simulink library "ECO_TestLibs"  (R2018a)
settings: Solver=ode45  StartTime=0.0  StopTime=10.0  RelTol=1e-3  EnableMultiTasking=on
undefined symbols (not defined in the file or in its folder): h, km
libraries: CoderSF_BSW_Libs x643, $bdroot x217, SF_CanService_Libs x60, simulink x12
(part 7 of 7)

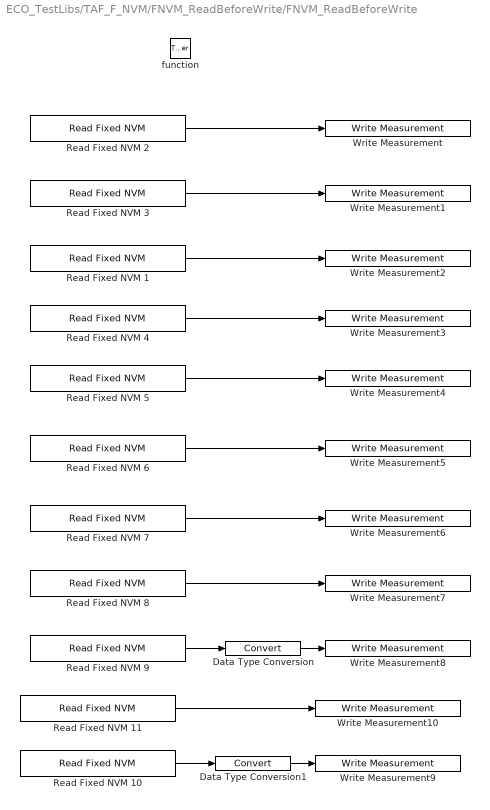
== system ECO_TestLibs/TAF_F_NVM/FNVM_ReadBeforeWrite/FNVM_ReadBeforeWrite ==
  function : TriggerPort  TriggerType=function-call  VariantControl=(inherit)
  Data Type Conversion : DataTypeConversion
  Data Type Conversion1 : DataTypeConversion
  Read Fixed NVM 1 : CoderSF_BSW_Libs/Non-volatile Memory Blocks/Read Fixed NVM   data_name=Fnvm_single
      settings: SourceProductName=EcoCoder Blocks
  Read Fixed NVM 10 : CoderSF_BSW_Libs/Non-volatile Memory Blocks/Read Fixed NVM   data_name=Fnvm_double2
      settings: SourceProductName=EcoCoder Blocks
  Read Fixed NVM 11 : CoderSF_BSW_Libs/Non-volatile Memory Blocks/Read Fixed NVM   data_name=Fnvm_single2
      settings: SourceProductName=EcoCoder Blocks
  Read Fixed NVM 2 : CoderSF_BSW_Libs/Non-volatile Memory Blocks/Read Fixed NVM   data_name=Fnvm_int32
      settings: SourceProductName=EcoCoder Blocks
  Read Fixed NVM 3 : CoderSF_BSW_Libs/Non-volatile Memory Blocks/Read Fixed NVM   data_name=Fnvm_uint32
      settings: SourceProductName=EcoCoder Blocks
  Read Fixed NVM 4 : CoderSF_BSW_Libs/Non-volatile Memory Blocks/Read Fixed NVM   data_name=Fnvm_int16
      settings: SourceProductName=EcoCoder Blocks
  Read Fixed NVM 5 : CoderSF_BSW_Libs/Non-volatile Memory Blocks/Read Fixed NVM   data_name=Fnvm_uint16
      settings: SourceProductName=EcoCoder Blocks
  Read Fixed NVM 6 : CoderSF_BSW_Libs/Non-volatile Memory Blocks/Read Fixed NVM   data_name=Fnvm_boolean
      settings: SourceProductName=EcoCoder Blocks
  Read Fixed NVM 7 : CoderSF_BSW_Libs/Non-volatile Memory Blocks/Read Fixed NVM   data_name=Fnvm_uint8
      settings: SourceProductName=EcoCoder Blocks
  Read Fixed NVM 8 : CoderSF_BSW_Libs/Non-volatile Memory Blocks/Read Fixed NVM   data_name=Fnvm_int8
      settings: SourceProductName=EcoCoder Blocks
  Read Fixed NVM 9 : CoderSF_BSW_Libs/Non-volatile Memory Blocks/Read Fixed NVM   data_name=Fnvm_double
      settings: SourceProductName=EcoCoder Blocks
  Write Measurement : CoderSF_BSW_Libs/Calibration & Measurement/Write Measurement  variable_name=Fnvm_int32Init  variable_value=0  variable_type=int32  numD=1  unitStr=""  descStr=""
      settings: AttributesFormatString=value:%<variable_value> type:%<variable_type>  SourceProductName=EcoCoder Blocks
  Write Measurement1 : CoderSF_BSW_Libs/Calibration & Measurement/Write Measurement  variable_name=Fnvm_uint32Init  variable_value=0  variable_type=uint32  numD=4  unitStr=""  descStr=""
      settings: AttributesFormatString=value:%<variable_value> type:%<variable_type>  SourceProductName=EcoCoder Blocks
  Write Measurement10 : CoderSF_BSW_Libs/Calibration & Measurement/Write Measurement  variable_name=Fnvm_single2Init  variable_value=0  variable_type=single  numD=1  unitStr=""  descStr=""
      settings: AttributesFormatString=value:%<variable_value> type:%<variable_type>  SourceProductName=EcoCoder Blocks
  Write Measurement2 : CoderSF_BSW_Libs/Calibration & Measurement/Write Measurement  variable_name=Fnvm_singleInit  variable_value=0  variable_type=single  numD=1  unitStr=""  descStr=""
      settings: AttributesFormatString=value:%<variable_value> type:%<variable_type>  SourceProductName=EcoCoder Blocks
  Write Measurement3 : CoderSF_BSW_Libs/Calibration & Measurement/Write Measurement  variable_name=Fnvm_int16Init  variable_value=0  variable_type=int16  numD=2  unitStr=""  descStr=""
      settings: AttributesFormatString=value:%<variable_value> type:%<variable_type>  SourceProductName=EcoCoder Blocks
  Write Measurement4 : CoderSF_BSW_Libs/Calibration & Measurement/Write Measurement  variable_name=Fnvm_uint16Init  variable_value=0  variable_type=uint16  numD=2  unitStr=""  descStr=""
      settings: AttributesFormatString=value:%<variable_value> type:%<variable_type>  SourceProductName=EcoCoder Blocks
  Write Measurement5 : CoderSF_BSW_Libs/Calibration & Measurement/Write Measurement  variable_name=Fnvm_booleanInit  variable_value=0  variable_type=boolean  numD=4  unitStr=""  descStr=""
      settings: AttributesFormatString=value:%<variable_value> type:%<variable_type>  SourceProductName=EcoCoder Blocks
  Write Measurement6 : CoderSF_BSW_Libs/Calibration & Measurement/Write Measurement  variable_name=Fnvm_uint8Init  variable_value=0  variable_type=uint8  numD=1  unitStr=""  descStr=""
      settings: AttributesFormatString=value:%<variable_value> type:%<variable_type>  SourceProductName=EcoCoder Blocks
  Write Measurement7 : CoderSF_BSW_Libs/Calibration & Measurement/Write Measurement  variable_name=Fnvm_int8Init  variable_value=0  variable_type=int8  numD=2  unitStr=""  descStr=""
      settings: AttributesFormatString=value:%<variable_value> type:%<variable_type>  SourceProductName=EcoCoder Blocks
  Write Measurement8 : CoderSF_BSW_Libs/Calibration & Measurement/Write Measurement  variable_name=Fnvm_doubleInit  variable_value=0  variable_type=single  numD=1  unitStr=""  descStr=""
      settings: AttributesFormatString=value:%<variable_value> type:%<variable_type>  SourceProductName=EcoCoder Blocks
  Write Measurement9 : CoderSF_BSW_Libs/Calibration & Measurement/Write Measurement  variable_name=Fnvm_double2Init  variable_value=0  variable_type=single  numD=1  unitStr=""  descStr=""
      settings: AttributesFormatString=value:%<variable_value> type:%<variable_type>  SourceProductName=EcoCoder Blocks
  wires:
  Read Fixed NVM 8/1 -> Write Measurement7/1
  Read Fixed NVM 6/1 -> Write Measurement5/1
  Read Fixed NVM 5/1 -> Write Measurement4/1
  Read Fixed NVM 1/1 -> Write Measurement2/1
  Read Fixed NVM 9/1 -> Data Type Conversion/1
  Read Fixed NVM 3/1 -> Write Measurement1/1
  Read Fixed NVM 4/1 -> Write Measurement3/1
  Data Type Conversion/1 -> Write Measurement8/1
  Read Fixed NVM 2/1 -> Write Measurement/1
  Read Fixed NVM 7/1 -> Write Measurement6/1
  Read Fixed NVM 10/1 -> Data Type Conversion1/1
  Data Type Conversion1/1 -> Write Measurement9/1
  Read Fixed NVM 11/1 -> Write Measurement10/1

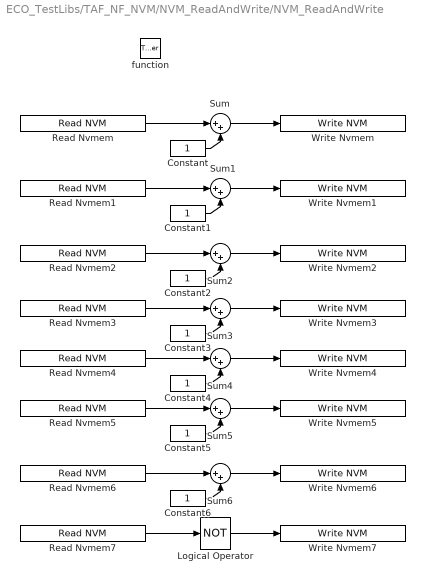
== system ECO_TestLibs/TAF_NF_NVM/NVM_ReadAndWrite/NVM_ReadAndWrite ==
  function : TriggerPort  TriggerType=function-call  VariantControl=(inherit)
  Constant{,1..6} (7 alike) : Constant  OutDataTypeStr=Inherit: Inherit via back propagation  SampleTime=-1
  Logical Operator : Logic  Operator=NOT  AllPortsSameDT=off  OutDataTypeStr=boolean
  Read Nvmem : CoderSF_BSW_Libs/Non-volatile Memory Blocks/Read NVM  variable_name=ASW_Nvm_single  variable_type=Inherit from 'Variable definition'
      settings: AttributesFormatString=type:%<variable_type>  SourceProductName=EcoCoder Blocks
  Read Nvmem1 : CoderSF_BSW_Libs/Non-volatile Memory Blocks/Read NVM  variable_name=ASW_Nvm_int8  variable_type=Inherit from 'Variable definition'
      settings: AttributesFormatString=type:%<variable_type>  SourceProductName=EcoCoder Blocks
  Read Nvmem2 : CoderSF_BSW_Libs/Non-volatile Memory Blocks/Read NVM  variable_name=ASW_Nvm_uint8  variable_type=Inherit from 'Variable definition'
      settings: AttributesFormatString=type:%<variable_type>  SourceProductName=EcoCoder Blocks
  Read Nvmem3 : CoderSF_BSW_Libs/Non-volatile Memory Blocks/Read NVM  variable_name=ASW_Nvm_int16  variable_type=Inherit from 'Variable definition'
      settings: AttributesFormatString=type:%<variable_type>  SourceProductName=EcoCoder Blocks
  Read Nvmem4 : CoderSF_BSW_Libs/Non-volatile Memory Blocks/Read NVM  variable_name=ASW_Nvm_uint16  variable_type=Inherit from 'Variable definition'
      settings: AttributesFormatString=type:%<variable_type>  SourceProductName=EcoCoder Blocks
  Read Nvmem5 : CoderSF_BSW_Libs/Non-volatile Memory Blocks/Read NVM  variable_name=ASW_Nvm_int32  variable_type=Inherit from 'Variable definition'
      settings: AttributesFormatString=type:%<variable_type>  SourceProductName=EcoCoder Blocks
  Read Nvmem6 : CoderSF_BSW_Libs/Non-volatile Memory Blocks/Read NVM  variable_name=ASW_Nvm_uint32  variable_type=Inherit from 'Variable definition'
      settings: AttributesFormatString=type:%<variable_type>  SourceProductName=EcoCoder Blocks
  Read Nvmem7 : CoderSF_BSW_Libs/Non-volatile Memory Blocks/Read NVM  variable_name=ASW_Nvm_boolean  variable_type=Inherit from 'Variable definition'
      settings: AttributesFormatString=type:%<variable_type>  SourceProductName=EcoCoder Blocks
  Sum{,1..6} (7 alike) : Sum  Inputs=|++
  Write Nvmem : CoderSF_BSW_Libs/Non-volatile Memory Blocks/Write NVM  variable_name=ASW_Nvm_single  flgDef=on  variable_value=2  variable_type=single  variable_numD=1  unitStr=""  descStr=""  EcoCoderBlockID=N001_NVMVDEF
      settings: AttributesFormatString=value:%<variable_value> type:%<variable_type> D:%<variable_numD>  SourceProductName=EcoCoder Blocks
  Write Nvmem1 : CoderSF_BSW_Libs/Non-volatile Memory Blocks/Write NVM  variable_name=ASW_Nvm_int8  flgDef=on  variable_value=2  variable_type=int8  variable_numD=1  unitStr=""  descStr=""  EcoCoderBlockID=N001_NVMVDEF
      settings: AttributesFormatString=value:%<variable_value> type:%<variable_type> D:%<variable_numD>  SourceProductName=EcoCoder Blocks
  Write Nvmem2 : CoderSF_BSW_Libs/Non-volatile Memory Blocks/Write NVM  variable_name=ASW_Nvm_uint8  flgDef=on  variable_value=2  variable_type=uint8  variable_numD=1  unitStr=""  descStr=""  EcoCoderBlockID=N001_NVMVDEF
      settings: AttributesFormatString=value:%<variable_value> type:%<variable_type> D:%<variable_numD>  SourceProductName=EcoCoder Blocks
  Write Nvmem3 : CoderSF_BSW_Libs/Non-volatile Memory Blocks/Write NVM  variable_name=ASW_Nvm_int16  flgDef=on  variable_value=2  variable_type=int16  variable_numD=1  unitStr=""  descStr=""  EcoCoderBlockID=N001_NVMVDEF
      settings: AttributesFormatString=value:%<variable_value> type:%<variable_type> D:%<variable_numD>  SourceProductName=EcoCoder Blocks
  Write Nvmem4 : CoderSF_BSW_Libs/Non-volatile Memory Blocks/Write NVM  variable_name=ASW_Nvm_uint16  flgDef=on  variable_value=2  variable_type=uint16  variable_numD=1  unitStr=""  descStr=""  EcoCoderBlockID=N001_NVMVDEF
      settings: AttributesFormatString=value:%<variable_value> type:%<variable_type> D:%<variable_numD>  SourceProductName=EcoCoder Blocks
  Write Nvmem5 : CoderSF_BSW_Libs/Non-volatile Memory Blocks/Write NVM  variable_name=ASW_Nvm_int32  flgDef=on  variable_value=2  variable_type=int32  variable_numD=1  unitStr=""  descStr=""  EcoCoderBlockID=N001_NVMVDEF
      settings: AttributesFormatString=value:%<variable_value> type:%<variable_type> D:%<variable_numD>  SourceProductName=EcoCoder Blocks
  Write Nvmem6 : CoderSF_BSW_Libs/Non-volatile Memory Blocks/Write NVM  variable_name=ASW_Nvm_uint32  flgDef=on  variable_value=2  variable_type=uint32  variable_numD=1  unitStr=""  descStr=""  EcoCoderBlockID=N001_NVMVDEF
      settings: AttributesFormatString=value:%<variable_value> type:%<variable_type> D:%<variable_numD>  SourceProductName=EcoCoder Blocks
  Write Nvmem7 : CoderSF_BSW_Libs/Non-volatile Memory Blocks/Write NVM  variable_name=ASW_Nvm_boolean  flgDef=on  variable_value=0  variable_type=boolean  variable_numD=1  unitStr=""  descStr=""  EcoCoderBlockID=N001_NVMVDEF
      settings: AttributesFormatString=value:%<variable_value> type:%<variable_type> D:%<variable_numD>  SourceProductName=EcoCoder Blocks
  wires:
  Read Nvmem7/1 -> Logical Operator/1
  Logical Operator/1 -> Write Nvmem7/1
  Read Nvmem6/1 -> Sum6/1
  Constant6/1 -> Sum6/2
  Sum6/1 -> Write Nvmem6/1
  Read Nvmem5/1 -> Sum5/1
  Constant5/1 -> Sum5/2
  Sum5/1 -> Write Nvmem5/1
  Read Nvmem4/1 -> Sum4/1
  Constant4/1 -> Sum4/2
  Sum4/1 -> Write Nvmem4/1
  Read Nvmem3/1 -> Sum3/1
  Constant3/1 -> Sum3/2
  Sum3/1 -> Write Nvmem3/1
  Read Nvmem2/1 -> Sum2/1
  Constant2/1 -> Sum2/2
  Sum2/1 -> Write Nvmem2/1
  Read Nvmem1/1 -> Sum1/1
  Constant1/1 -> Sum1/2
  Sum1/1 -> Write Nvmem1/1
  Read Nvmem/1 -> Sum/1
  Constant/1 -> Sum/2
  Sum/1 -> Write Nvmem/1

== system ECO_TestLibs/TAF_NF_NVM/NVM_ReadBeforeWrite/NVM_ReadBeforeWrite ==
  function : TriggerPort  TriggerType=function-call  VariantControl=(inherit)
  Measurement Probe : CoderSF_BSW_Libs/Calibration & Measurement/Write Measurement  variable_name=ASW_V_singleInit  variable_value=0  variable_type=single  numD=1  unitStr=""  descStr=""
      settings: AttributesFormatString=value:%<variable_value> type:%<variable_type>  SourceProductName=EcoCoder Blocks
  Measurement Probe1 : CoderSF_BSW_Libs/Calibration & Measurement/Write Measurement  variable_name=ASW_V_int8Init  variable_value=0  variable_type=int8  numD=1  unitStr=""  descStr=""
      settings: AttributesFormatString=value:%<variable_value> type:%<variable_type>  SourceProductName=EcoCoder Blocks
  Measurement Probe2 : CoderSF_BSW_Libs/Calibration & Measurement/Write Measurement  variable_name=ASW_V_uint8Init  variable_value=0  variable_type=uint8  numD=1  unitStr=""  descStr=""
      settings: AttributesFormatString=value:%<variable_value> type:%<variable_type>  SourceProductName=EcoCoder Blocks
  Measurement Probe3 : CoderSF_BSW_Libs/Calibration & Measurement/Write Measurement  variable_name=ASW_V_int16Init  variable_value=0  variable_type=int16  numD=1  unitStr=""  descStr=""
      settings: AttributesFormatString=value:%<variable_value> type:%<variable_type>  SourceProductName=EcoCoder Blocks
  Measurement Probe4 : CoderSF_BSW_Libs/Calibration & Measurement/Write Measurement  variable_name=ASW_V_uint16Init  variable_value=0  variable_type=uint16  numD=1  unitStr=""  descStr=""
      settings: AttributesFormatString=value:%<variable_value> type:%<variable_type>  SourceProductName=EcoCoder Blocks
  Measurement Probe5 : CoderSF_BSW_Libs/Calibration & Measurement/Write Measurement  variable_name=ASW_V_int32Init  variable_value=0  variable_type=int32  numD=1  unitStr=""  descStr=""
      settings: AttributesFormatString=value:%<variable_value> type:%<variable_type>  SourceProductName=EcoCoder Blocks
  Measurement Probe6 : CoderSF_BSW_Libs/Calibration & Measurement/Write Measurement  variable_name=ASW_V_uint32Init  variable_value=0  variable_type=uint32  numD=1  unitStr=""  descStr=""
      settings: AttributesFormatString=value:%<variable_value> type:%<variable_type>  SourceProductName=EcoCoder Blocks
  Measurement Probe7 : CoderSF_BSW_Libs/Calibration & Measurement/Write Measurement  variable_name=ASW_V_booleanInit  variable_value=0  variable_type=boolean  numD=1  unitStr=""  descStr=""
      settings: AttributesFormatString=value:%<variable_value> type:%<variable_type>  SourceProductName=EcoCoder Blocks
  Read Nvmem : CoderSF_BSW_Libs/Non-volatile Memory Blocks/Read NVM  variable_name=ASW_Nvm_single  variable_type=Inherit from 'Variable definition'
      settings: AttributesFormatString=type:%<variable_type>  SourceProductName=EcoCoder Blocks
  Read Nvmem1 : CoderSF_BSW_Libs/Non-volatile Memory Blocks/Read NVM  variable_name=ASW_Nvm_int8  variable_type=Inherit from 'Variable definition'
      settings: AttributesFormatString=type:%<variable_type>  SourceProductName=EcoCoder Blocks
  Read Nvmem2 : CoderSF_BSW_Libs/Non-volatile Memory Blocks/Read NVM  variable_name=ASW_Nvm_uint8  variable_type=Inherit from 'Variable definition'
      settings: AttributesFormatString=type:%<variable_type>  SourceProductName=EcoCoder Blocks
  Read Nvmem3 : CoderSF_BSW_Libs/Non-volatile Memory Blocks/Read NVM  variable_name=ASW_Nvm_int16  variable_type=Inherit from 'Variable definition'
      settings: AttributesFormatString=type:%<variable_type>  SourceProductName=EcoCoder Blocks
  Read Nvmem4 : CoderSF_BSW_Libs/Non-volatile Memory Blocks/Read NVM  variable_name=ASW_Nvm_uint16  variable_type=Inherit from 'Variable definition'
      settings: AttributesFormatString=type:%<variable_type>  SourceProductName=EcoCoder Blocks
  Read Nvmem5 : CoderSF_BSW_Libs/Non-volatile Memory Blocks/Read NVM  variable_name=ASW_Nvm_int32  variable_type=Inherit from 'Variable definition'
      settings: AttributesFormatString=type:%<variable_type>  SourceProductName=EcoCoder Blocks
  Read Nvmem6 : CoderSF_BSW_Libs/Non-volatile Memory Blocks/Read NVM  variable_name=ASW_Nvm_uint32  variable_type=Inherit from 'Variable definition'
      settings: AttributesFormatString=type:%<variable_type>  SourceProductName=EcoCoder Blocks
  Read Nvmem7 : CoderSF_BSW_Libs/Non-volatile Memory Blocks/Read NVM  variable_name=ASW_Nvm_boolean  variable_type=Inherit from 'Variable definition'
      settings: AttributesFormatString=type:%<variable_type>  SourceProductName=EcoCoder Blocks
  wires:
  Read Nvmem/1 -> Measurement Probe/1
  Read Nvmem1/1 -> Measurement Probe1/1
  Read Nvmem2/1 -> Measurement Probe2/1
  Read Nvmem3/1 -> Measurement Probe3/1
  Read Nvmem4/1 -> Measurement Probe4/1
  Read Nvmem5/1 -> Measurement Probe5/1
  Read Nvmem6/1 -> Measurement Probe6/1
  Read Nvmem7/1 -> Measurement Probe7/1

== system ECO_TestLibs/TAF_NF_NVM/Test_NVMStoreFailed/F_Store_All_NVM_Data ==
  function : TriggerPort  TriggerType=function-call  VariantControl=(inherit)
  Logical Operator : Logic  Operator=NOT  AllPortsSameDT=off  OutDataTypeStr=boolean
  Store All NVM Data : CoderSF_BSW_Libs/Non-volatile Memory Blocks/Store All NVM Data  TriggerTypeSet=rising
      settings: SourceProductName=EcoCoder Blocks
  Unit Delay : UnitDelay  SampleTime=-1
  wires:
  Logical Operator/1 -> Unit Delay/1
  Unit Delay/1 -> Store All NVM Data/Trigger, Logical Operator/1

== system ECO_TestLibs/TAF_SWD/TAF_SWD/Service Software Watchdog ==
  Enable : EnablePort
  Service Software Watchdog : CoderSF_BSW_Libs/System Management Blocks/Service Software Watchdog  EcoCoderBlockID=W001_WDGFeed
      settings: SourceProductName=EcoCoder Blocks

== system ECO_TestLibs/TAF_SYS/Shutdown Power/Enabled Subsystem ==
  Enable : EnablePort
  Read Calibration2 : CoderSF_BSW_Libs/Calibration & Measurement/Read Calibration  variable_name=WKUP_flgPwrDelay_val  variable_value=0  variable_type=boolean  variable_min=[]  variable_max=[]  unitStr=""  descStr=""
      settings: AttributesFormatString=value:%<variable_value> type:%<variable_type> max:%<variable_max> Min:%<variable_min>  SourceProductName=EcoCoder Blocks
  "Switch Internal " : CoderSF_BSW_Libs/Digital I//O/Switch Internal   portNum=PowerDelay
      settings: SourceProductName=EcoCoder Blocks
  Write and Read Measurement2 : CoderSF_BSW_Libs/Calibration & Measurement/Write and Read Measurement  variable_name=WKUP_flgPwrDelay  variable_value=0  variable_type=boolean  numD=1  unitStr=""  descStr=""
      settings: AttributesFormatString=value:%<variable_value> type:%<variable_type>  SourceProductName=EcoCoder Blocks
  wires:
  Read Calibration2/1 -> Write and Read Measurement2/1
  Write and Read Measurement2/1 -> "Switch Internal "/1

== system ECO_TestLibs/TAF_TRI/Test_DeadWhile_H1m/Function-Call Subsystem ==
  In1 : Inport
  function : TriggerPort  TriggerType=function-call  VariantControl=(inherit)
  Out1 : Outport
  wires:
  In1/1 -> Out1/1

== system ECO_TestLibs/TAF_TRI/Test_DeadWhile_L1m/Function-Call Subsystem ==
  In1 : Inport
  function : TriggerPort  TriggerType=function-call  VariantControl=(inherit)
  Out1 : Outport
  wires:
  In1/1 -> Out1/1

== system ECO_TestLibs/LINAMaster/RTX/Delay2/Rising Edge ==
  in : Inport  OutDataTypeStr=boolean
  Logical Operator : Logic  AllPortsSameDT=off  OutDataTypeStr=boolean
  Logical Operator1 : Logic  Operator=NOT  AllPortsSameDT=off  OutDataTypeStr=boolean
  Unit Delay : UnitDelay  InitialCondition=InitialCondition  SampleTime=-1
  out : Outport  OutDataTypeStr=boolean
  wires:
  Logical Operator1/1 -> Logical Operator/2
  Logical Operator/1 -> out/1
  Unit Delay/1 -> Logical Operator1/1
  in/1 -> Unit Delay/1, Logical Operator/1

== system ECO_TestLibs/LINAMaster/RTX/Mst Rx Mod/Subsystem ==
  In1 : Inport
  Trigger : TriggerPort  VariantControl=(inherit)  PortDimensions=1
  Send CAN Data : CoderSF_BSW_Libs/CAN/Send CAN Data  channel=CAN_C  txlen=3  txid=hex2dec('200')  frametype=Standard(11-bit ID)  showerror=off
      settings: SourceProductName=EcoCoder Blocks
  wires:
  In1/1 -> Send CAN Data/1

== system ECO_TestLibs/LINASlave/Rx/Subsystem/cntValue1 ==
  10 : Constant  Value=10  OutDataTypeStr=Inherit: Inherit via back propagation
  5 : Constant  Value=1000000000  OutDataTypeStr=Inherit: Inherit via back propagation
  6 : Constant  OutDataTypeStr=Inherit: Inherit via back propagation
  7 : Constant  Value=10000000  OutDataTypeStr=Inherit: Inherit via back propagation
  8 : Constant  Value=100000  OutDataTypeStr=Inherit: Inherit via back propagation
  9 : Constant  Value=1000  OutDataTypeStr=Inherit: Inherit via back propagation
  Delay : simulink/Discrete/Integer Delay  NumDelays=1  vinit=1  samptime=-1
      settings: SourceProductName=Simulink  SourceProductBaseCode=SL
  Sum : Sum  Inputs=|++
  Terminator : Terminator
  ValueConvert : Subsystem
  ValueConvert1 : Subsystem
  ValueConvert2 : Subsystem
  ValueConvert3 : Subsystem
  ValueConvert4 : Subsystem
  m0 : CoderSF_BSW_Libs/Calibration & Measurement/Write and Read Measurement  variable_name=cnt0  variable_value=0  variable_type=uint32  numD=1  unitStr=""  descStr=""
      settings: AttributesFormatString=type:%<variable_type> Dimensions:%<numD>  SourceProductName=EcoCoder Blocks
  Out1 : Outport
  Out2 : Outport  Port=2
  Out3 : Outport  Port=3
  Out4 : Outport  Port=4
  Out5 : Outport  Port=5
  wires:
  ValueConvert/1(Out1) -> Out1/1
  5/1 -> ValueConvert/2(In2)
  7/1 -> ValueConvert1/2(In2)
  8/1 -> ValueConvert2/2(In2)
  9/1 -> ValueConvert3/2(In2)
  10/1 -> ValueConvert4/2(In2)
  m0/1 -> ValueConvert/1(In1)
  6/1 -> Sum/2
  Delay/1 -> Sum/1, m0/1
  Sum/1 -> Delay/1
  ValueConvert1/1(Out1) -> Out2/1
  ValueConvert/2(Out2) -> ValueConvert1/1(In1)
  ValueConvert1/2(Out2) -> ValueConvert2/1(In1)
  ValueConvert2/1(Out1) -> Out3/1
  ValueConvert2/2(Out2) -> ValueConvert3/1(In1)
  ValueConvert3/1(Out1) -> Out4/1
  ValueConvert3/2(Out2) -> ValueConvert4/1(In1)
  ValueConvert4/1(Out1) -> Out5/1
  ValueConvert4/2(Out2) -> Terminator/1

== system ECO_TestLibs/LINASlave/Rx/Subsystem1/cntValue1 ==
  10 : Constant  Value=10  OutDataTypeStr=Inherit: Inherit via back propagation
  5 : Constant  Value=1000000000  OutDataTypeStr=Inherit: Inherit via back propagation
  6 : Constant  OutDataTypeStr=Inherit: Inherit via back propagation
  7 : Constant  Value=10000000  OutDataTypeStr=Inherit: Inherit via back propagation
  8 : Constant  Value=100000  OutDataTypeStr=Inherit: Inherit via back propagation
  9 : Constant  Value=1000  OutDataTypeStr=Inherit: Inherit via back propagation
  Delay : simulink/Discrete/Integer Delay  NumDelays=1  vinit=1  samptime=-1
      settings: SourceProductName=Simulink  SourceProductBaseCode=SL
  Sum : Sum  Inputs=|++
  Terminator : Terminator
  ValueConvert : Subsystem
  ValueConvert1 : Subsystem
  ValueConvert2 : Subsystem
  ValueConvert3 : Subsystem
  ValueConvert4 : Subsystem
  m0 : CoderSF_BSW_Libs/Calibration & Measurement/Write and Read Measurement  variable_name=cnt1  variable_value=0  variable_type=uint32  numD=1  unitStr=""  descStr=""
      settings: AttributesFormatString=type:%<variable_type> Dimensions:%<numD>  SourceProductName=EcoCoder Blocks
  Out1 : Outport
  Out2 : Outport  Port=2
  Out3 : Outport  Port=3
  Out4 : Outport  Port=4
  Out5 : Outport  Port=5
  wires:
  ValueConvert/1(Out1) -> Out1/1
  5/1 -> ValueConvert/2(In2)
  7/1 -> ValueConvert1/2(In2)
  8/1 -> ValueConvert2/2(In2)
  9/1 -> ValueConvert3/2(In2)
  10/1 -> ValueConvert4/2(In2)
  m0/1 -> ValueConvert/1(In1)
  6/1 -> Sum/2
  Delay/1 -> Sum/1, m0/1
  Sum/1 -> Delay/1
  ValueConvert1/1(Out1) -> Out2/1
  ValueConvert/2(Out2) -> ValueConvert1/1(In1)
  ValueConvert1/2(Out2) -> ValueConvert2/1(In1)
  ValueConvert2/1(Out1) -> Out3/1
  ValueConvert2/2(Out2) -> ValueConvert3/1(In1)
  ValueConvert3/1(Out1) -> Out4/1
  ValueConvert3/2(Out2) -> ValueConvert4/1(In1)
  ValueConvert4/1(Out1) -> Out5/1
  ValueConvert4/2(Out2) -> Terminator/1

== system ECO_TestLibs/LINASlave/Rx/Subsystem2/cntValue ==
  10 : Constant  Value=10  OutDataTypeStr=Inherit: Inherit via back propagation
  5 : Constant  Value=1000000000  OutDataTypeStr=Inherit: Inherit via back propagation
  6 : Constant  OutDataTypeStr=Inherit: Inherit via back propagation
  7 : Constant  Value=10000000  OutDataTypeStr=Inherit: Inherit via back propagation
  8 : Constant  Value=100000  OutDataTypeStr=Inherit: Inherit via back propagation
  9 : Constant  Value=1000  OutDataTypeStr=Inherit: Inherit via back propagation
  Delay : simulink/Discrete/Integer Delay  NumDelays=1  vinit=1  samptime=-1
      settings: SourceProductName=Simulink  SourceProductBaseCode=SL
  Sum : Sum  Inputs=|++
  Terminator : Terminator
  ValueConvert : Subsystem
  ValueConvert1 : Subsystem
  ValueConvert2 : Subsystem
  ValueConvert3 : Subsystem
  ValueConvert4 : Subsystem
  m0 : CoderSF_BSW_Libs/Calibration & Measurement/Write and Read Measurement  variable_name=cnt2  variable_value=0  variable_type=uint32  numD=1  unitStr=""  descStr=""
      settings: AttributesFormatString=type:%<variable_type> Dimensions:%<numD>  SourceProductName=EcoCoder Blocks
  Out1 : Outport
  Out2 : Outport  Port=2
  Out3 : Outport  Port=3
  Out4 : Outport  Port=4
  Out5 : Outport  Port=5
  wires:
  ValueConvert/1(Out1) -> Out1/1
  5/1 -> ValueConvert/2(In2)
  7/1 -> ValueConvert1/2(In2)
  8/1 -> ValueConvert2/2(In2)
  9/1 -> ValueConvert3/2(In2)
  10/1 -> ValueConvert4/2(In2)
  m0/1 -> ValueConvert/1(In1)
  6/1 -> Sum/2
  Delay/1 -> Sum/1, m0/1
  Sum/1 -> Delay/1
  ValueConvert1/1(Out1) -> Out2/1
  ValueConvert/2(Out2) -> ValueConvert1/1(In1)
  ValueConvert1/2(Out2) -> ValueConvert2/1(In1)
  ValueConvert2/1(Out1) -> Out3/1
  ValueConvert2/2(Out2) -> ValueConvert3/1(In1)
  ValueConvert3/1(Out1) -> Out4/1
  ValueConvert3/2(Out2) -> ValueConvert4/1(In1)
  ValueConvert4/1(Out1) -> Out5/1
  ValueConvert4/2(Out2) -> Terminator/1

== system ECO_TestLibs/LINASlave/Rx/Subsystem/cntValue1/ValueConvert ==
  In1 : Inport
  In2 : Inport  Port=2
  1 : Constant  Value=10  OutDataTypeStr=Inherit: Inherit via back propagation
  7 : Constant  Value=16  OutDataTypeStr=Inherit: Inherit via back propagation
  Data Type Conversion : DataTypeConversion
  Divide : Product  Inputs=*/
  Divide1 : Product  Inputs=**
  Divide2 : Product  Inputs=*/
  Divide3 : Product  Inputs=*/
  Math Function : Math  Operator=mod  SaturateOnIntegerOverflow=on
  Math Function1 : Math  Operator=mod  SaturateOnIntegerOverflow=on
  Sum1 : Sum  Inputs=|++
  Out1 : Outport
  Out2 : Outport  Port=2
  wires:
  Divide2/1 -> Sum1/2
  7/1 -> Divide1/2
  Divide1/1 -> Sum1/1
  Math Function/1 -> Divide2/1, Math Function1/1
  Sum1/1 -> Data Type Conversion/1
  [ModeValue] -> Math Function/2
  [ModeValue] -> Divide/2
  Divide/1 -> Divide1/1
  In2/1 -> [ModeValue]
  [ModeValue] -> Divide3/1
  Divide3/1 -> Math Function1/2, Divide2/2
  1/1 -> Divide3/2
  Data Type Conversion/1 -> Out1/1
  In1/1 -> Math Function/1, Divide/1
  Math Function1/1 -> Out2/1

== system ECO_TestLibs/LINASlave/Rx/Subsystem/cntValue1/ValueConvert1 ==
  In1 : Inport
  In2 : Inport  Port=2
  1 : Constant  Value=10  OutDataTypeStr=Inherit: Inherit via back propagation
  7 : Constant  Value=16  OutDataTypeStr=Inherit: Inherit via back propagation
  Data Type Conversion : DataTypeConversion
  Divide : Product  Inputs=*/
  Divide1 : Product  Inputs=**
  Divide2 : Product  Inputs=*/
  Divide3 : Product  Inputs=*/
  Math Function : Math  Operator=mod  SaturateOnIntegerOverflow=on
  Math Function1 : Math  Operator=mod  SaturateOnIntegerOverflow=on
  Sum1 : Sum  Inputs=|++
  Out1 : Outport
  Out2 : Outport  Port=2
  wires:
  Math Function1/1 -> Out2/1
  In1/1 -> Divide/1, Math Function/1
  Data Type Conversion/1 -> Out1/1
  1/1 -> Divide3/2
  Divide3/1 -> Divide2/2, Math Function1/2
  [ModeValue] -> Divide3/1
  In2/1 -> [ModeValue]
  Divide/1 -> Divide1/1
  [ModeValue] -> Divide/2
  [ModeValue] -> Math Function/2
  Sum1/1 -> Data Type Conversion/1
  Math Function/1 -> Math Function1/1, Divide2/1
  Divide1/1 -> Sum1/1
  7/1 -> Divide1/2
  Divide2/1 -> Sum1/2

== system ECO_TestLibs/LINASlave/Rx/Subsystem/cntValue1/ValueConvert2 ==
  In1 : Inport
  In2 : Inport  Port=2
  1 : Constant  Value=10  OutDataTypeStr=Inherit: Inherit via back propagation
  7 : Constant  Value=16  OutDataTypeStr=Inherit: Inherit via back propagation
  Data Type Conversion : DataTypeConversion
  Divide : Product  Inputs=*/
  Divide1 : Product  Inputs=**
  Divide2 : Product  Inputs=*/
  Divide3 : Product  Inputs=*/
  Math Function : Math  Operator=mod  SaturateOnIntegerOverflow=on
  Math Function1 : Math  Operator=mod  SaturateOnIntegerOverflow=on
  Sum1 : Sum  Inputs=|++
  Out1 : Outport
  Out2 : Outport  Port=2
  wires:
  Divide2/1 -> Sum1/2
  7/1 -> Divide1/2
  Divide1/1 -> Sum1/1
  Math Function/1 -> Divide2/1, Math Function1/1
  Sum1/1 -> Data Type Conversion/1
  [ModeValue] -> Math Function/2
  [ModeValue] -> Divide/2
  Divide/1 -> Divide1/1
  In2/1 -> [ModeValue]
  [ModeValue] -> Divide3/1
  Divide3/1 -> Math Function1/2, Divide2/2
  1/1 -> Divide3/2
  Data Type Conversion/1 -> Out1/1
  In1/1 -> Math Function/1, Divide/1
  Math Function1/1 -> Out2/1

== system ECO_TestLibs/LINASlave/Rx/Subsystem/cntValue1/ValueConvert3 ==
  In1 : Inport
  In2 : Inport  Port=2
  1 : Constant  Value=10  OutDataTypeStr=Inherit: Inherit via back propagation
  7 : Constant  Value=16  OutDataTypeStr=Inherit: Inherit via back propagation
  Data Type Conversion : DataTypeConversion
  Divide : Product  Inputs=*/
  Divide1 : Product  Inputs=**
  Divide2 : Product  Inputs=*/
  Divide3 : Product  Inputs=*/
  Math Function : Math  Operator=mod  SaturateOnIntegerOverflow=on
  Math Function1 : Math  Operator=mod  SaturateOnIntegerOverflow=on
  Sum1 : Sum  Inputs=|++
  Out1 : Outport
  Out2 : Outport  Port=2
  wires:
  Math Function1/1 -> Out2/1
  In1/1 -> Divide/1, Math Function/1
  Data Type Conversion/1 -> Out1/1
  1/1 -> Divide3/2
  Divide3/1 -> Divide2/2, Math Function1/2
  [ModeValue] -> Divide3/1
  In2/1 -> [ModeValue]
  Divide/1 -> Divide1/1
  [ModeValue] -> Divide/2
  [ModeValue] -> Math Function/2
  Sum1/1 -> Data Type Conversion/1
  Math Function/1 -> Math Function1/1, Divide2/1
  Divide1/1 -> Sum1/1
  7/1 -> Divide1/2
  Divide2/1 -> Sum1/2

== system ECO_TestLibs/LINASlave/Rx/Subsystem/cntValue1/ValueConvert4 ==
  In1 : Inport
  In2 : Inport  Port=2
  1 : Constant  Value=10  OutDataTypeStr=Inherit: Inherit via back propagation
  7 : Constant  Value=16  OutDataTypeStr=Inherit: Inherit via back propagation
  Data Type Conversion : DataTypeConversion
  Divide : Product  Inputs=*/
  Divide1 : Product  Inputs=**
  Divide2 : Product  Inputs=*/
  Divide3 : Product  Inputs=*/
  Math Function : Math  Operator=mod  SaturateOnIntegerOverflow=on
  Math Function1 : Math  Operator=mod  SaturateOnIntegerOverflow=on
  Sum1 : Sum  Inputs=|++
  Out1 : Outport
  Out2 : Outport  Port=2
  wires:
  Divide2/1 -> Sum1/2
  7/1 -> Divide1/2
  Divide1/1 -> Sum1/1
  Math Function/1 -> Divide2/1, Math Function1/1
  Sum1/1 -> Data Type Conversion/1
  [ModeValue] -> Math Function/2
  [ModeValue] -> Divide/2
  Divide/1 -> Divide1/1
  In2/1 -> [ModeValue]
  [ModeValue] -> Divide3/1
  Divide3/1 -> Math Function1/2, Divide2/2
  1/1 -> Divide3/2
  Data Type Conversion/1 -> Out1/1
  In1/1 -> Math Function/1, Divide/1
  Math Function1/1 -> Out2/1

== system ECO_TestLibs/LINASlave/Rx/Subsystem1/cntValue1/ValueConvert ==
  In1 : Inport
  In2 : Inport  Port=2
  1 : Constant  Value=10  OutDataTypeStr=Inherit: Inherit via back propagation
  7 : Constant  Value=16  OutDataTypeStr=Inherit: Inherit via back propagation
  Data Type Conversion : DataTypeConversion
  Divide : Product  Inputs=*/
  Divide1 : Product  Inputs=**
  Divide2 : Product  Inputs=*/
  Divide3 : Product  Inputs=*/
  Math Function : Math  Operator=mod  SaturateOnIntegerOverflow=on
  Math Function1 : Math  Operator=mod  SaturateOnIntegerOverflow=on
  Sum1 : Sum  Inputs=|++
  Out1 : Outport
  Out2 : Outport  Port=2
  wires:
  Divide2/1 -> Sum1/2
  7/1 -> Divide1/2
  Divide1/1 -> Sum1/1
  Math Function/1 -> Divide2/1, Math Function1/1
  Sum1/1 -> Data Type Conversion/1
  [ModeValue] -> Math Function/2
  [ModeValue] -> Divide/2
  Divide/1 -> Divide1/1
  In2/1 -> [ModeValue]
  [ModeValue] -> Divide3/1
  Divide3/1 -> Math Function1/2, Divide2/2
  1/1 -> Divide3/2
  Data Type Conversion/1 -> Out1/1
  In1/1 -> Math Function/1, Divide/1
  Math Function1/1 -> Out2/1

== system ECO_TestLibs/LINASlave/Rx/Subsystem1/cntValue1/ValueConvert1 ==
  In1 : Inport
  In2 : Inport  Port=2
  1 : Constant  Value=10  OutDataTypeStr=Inherit: Inherit via back propagation
  7 : Constant  Value=16  OutDataTypeStr=Inherit: Inherit via back propagation
  Data Type Conversion : DataTypeConversion
  Divide : Product  Inputs=*/
  Divide1 : Product  Inputs=**
  Divide2 : Product  Inputs=*/
  Divide3 : Product  Inputs=*/
  Math Function : Math  Operator=mod  SaturateOnIntegerOverflow=on
  Math Function1 : Math  Operator=mod  SaturateOnIntegerOverflow=on
  Sum1 : Sum  Inputs=|++
  Out1 : Outport
  Out2 : Outport  Port=2
  wires:
  Math Function1/1 -> Out2/1
  In1/1 -> Divide/1, Math Function/1
  Data Type Conversion/1 -> Out1/1
  1/1 -> Divide3/2
  Divide3/1 -> Divide2/2, Math Function1/2
  [ModeValue] -> Divide3/1
  In2/1 -> [ModeValue]
  Divide/1 -> Divide1/1
  [ModeValue] -> Divide/2
  [ModeValue] -> Math Function/2
  Sum1/1 -> Data Type Conversion/1
  Math Function/1 -> Math Function1/1, Divide2/1
  Divide1/1 -> Sum1/1
  7/1 -> Divide1/2
  Divide2/1 -> Sum1/2

== system ECO_TestLibs/LINASlave/Rx/Subsystem1/cntValue1/ValueConvert2 ==
  In1 : Inport
  In2 : Inport  Port=2
  1 : Constant  Value=10  OutDataTypeStr=Inherit: Inherit via back propagation
  7 : Constant  Value=16  OutDataTypeStr=Inherit: Inherit via back propagation
  Data Type Conversion : DataTypeConversion
  Divide : Product  Inputs=*/
  Divide1 : Product  Inputs=**
  Divide2 : Product  Inputs=*/
  Divide3 : Product  Inputs=*/
  Math Function : Math  Operator=mod  SaturateOnIntegerOverflow=on
  Math Function1 : Math  Operator=mod  SaturateOnIntegerOverflow=on
  Sum1 : Sum  Inputs=|++
  Out1 : Outport
  Out2 : Outport  Port=2
  wires:
  Divide2/1 -> Sum1/2
  7/1 -> Divide1/2
  Divide1/1 -> Sum1/1
  Math Function/1 -> Divide2/1, Math Function1/1
  Sum1/1 -> Data Type Conversion/1
  [ModeValue] -> Math Function/2
  [ModeValue] -> Divide/2
  Divide/1 -> Divide1/1
  In2/1 -> [ModeValue]
  [ModeValue] -> Divide3/1
  Divide3/1 -> Math Function1/2, Divide2/2
  1/1 -> Divide3/2
  Data Type Conversion/1 -> Out1/1
  In1/1 -> Math Function/1, Divide/1
  Math Function1/1 -> Out2/1

== system ECO_TestLibs/LINASlave/Rx/Subsystem1/cntValue1/ValueConvert3 ==
  In1 : Inport
  In2 : Inport  Port=2
  1 : Constant  Value=10  OutDataTypeStr=Inherit: Inherit via back propagation
  7 : Constant  Value=16  OutDataTypeStr=Inherit: Inherit via back propagation
  Data Type Conversion : DataTypeConversion
  Divide : Product  Inputs=*/
  Divide1 : Product  Inputs=**
  Divide2 : Product  Inputs=*/
  Divide3 : Product  Inputs=*/
  Math Function : Math  Operator=mod  SaturateOnIntegerOverflow=on
  Math Function1 : Math  Operator=mod  SaturateOnIntegerOverflow=on
  Sum1 : Sum  Inputs=|++
  Out1 : Outport
  Out2 : Outport  Port=2
  wires:
  Math Function1/1 -> Out2/1
  In1/1 -> Divide/1, Math Function/1
  Data Type Conversion/1 -> Out1/1
  1/1 -> Divide3/2
  Divide3/1 -> Divide2/2, Math Function1/2
  [ModeValue] -> Divide3/1
  In2/1 -> [ModeValue]
  Divide/1 -> Divide1/1
  [ModeValue] -> Divide/2
  [ModeValue] -> Math Function/2
  Sum1/1 -> Data Type Conversion/1
  Math Function/1 -> Math Function1/1, Divide2/1
  Divide1/1 -> Sum1/1
  7/1 -> Divide1/2
  Divide2/1 -> Sum1/2

== system ECO_TestLibs/LINASlave/Rx/Subsystem1/cntValue1/ValueConvert4 ==
  In1 : Inport
  In2 : Inport  Port=2
  1 : Constant  Value=10  OutDataTypeStr=Inherit: Inherit via back propagation
  7 : Constant  Value=16  OutDataTypeStr=Inherit: Inherit via back propagation
  Data Type Conversion : DataTypeConversion
  Divide : Product  Inputs=*/
  Divide1 : Product  Inputs=**
  Divide2 : Product  Inputs=*/
  Divide3 : Product  Inputs=*/
  Math Function : Math  Operator=mod  SaturateOnIntegerOverflow=on
  Math Function1 : Math  Operator=mod  SaturateOnIntegerOverflow=on
  Sum1 : Sum  Inputs=|++
  Out1 : Outport
  Out2 : Outport  Port=2
  wires:
  Divide2/1 -> Sum1/2
  7/1 -> Divide1/2
  Divide1/1 -> Sum1/1
  Math Function/1 -> Divide2/1, Math Function1/1
  Sum1/1 -> Data Type Conversion/1
  [ModeValue] -> Math Function/2
  [ModeValue] -> Divide/2
  Divide/1 -> Divide1/1
  In2/1 -> [ModeValue]
  [ModeValue] -> Divide3/1
  Divide3/1 -> Math Function1/2, Divide2/2
  1/1 -> Divide3/2
  Data Type Conversion/1 -> Out1/1
  In1/1 -> Math Function/1, Divide/1
  Math Function1/1 -> Out2/1

== system ECO_TestLibs/LINASlave/Rx/Subsystem2/cntValue/ValueConvert ==
  In1 : Inport
  In2 : Inport  Port=2
  1 : Constant  Value=10  OutDataTypeStr=Inherit: Inherit via back propagation
  7 : Constant  Value=16  OutDataTypeStr=Inherit: Inherit via back propagation
  Data Type Conversion : DataTypeConversion
  Divide : Product  Inputs=*/
  Divide1 : Product  Inputs=**
  Divide2 : Product  Inputs=*/
  Divide3 : Product  Inputs=*/
  Math Function : Math  Operator=mod  SaturateOnIntegerOverflow=on
  Math Function1 : Math  Operator=mod  SaturateOnIntegerOverflow=on
  Sum1 : Sum  Inputs=|++
  Out1 : Outport
  Out2 : Outport  Port=2
  wires:
  Divide2/1 -> Sum1/2
  7/1 -> Divide1/2
  Divide1/1 -> Sum1/1
  Math Function/1 -> Divide2/1, Math Function1/1
  Sum1/1 -> Data Type Conversion/1
  [ModeValue] -> Math Function/2
  [ModeValue] -> Divide/2
  Divide/1 -> Divide1/1
  In2/1 -> [ModeValue]
  [ModeValue] -> Divide3/1
  Divide3/1 -> Math Function1/2, Divide2/2
  1/1 -> Divide3/2
  Data Type Conversion/1 -> Out1/1
  In1/1 -> Math Function/1, Divide/1
  Math Function1/1 -> Out2/1

== system ECO_TestLibs/LINASlave/Rx/Subsystem2/cntValue/ValueConvert1 ==
  In1 : Inport
  In2 : Inport  Port=2
  1 : Constant  Value=10  OutDataTypeStr=Inherit: Inherit via back propagation
  7 : Constant  Value=16  OutDataTypeStr=Inherit: Inherit via back propagation
  Data Type Conversion : DataTypeConversion
  Divide : Product  Inputs=*/
  Divide1 : Product  Inputs=**
  Divide2 : Product  Inputs=*/
  Divide3 : Product  Inputs=*/
  Math Function : Math  Operator=mod  SaturateOnIntegerOverflow=on
  Math Function1 : Math  Operator=mod  SaturateOnIntegerOverflow=on
  Sum1 : Sum  Inputs=|++
  Out1 : Outport
  Out2 : Outport  Port=2
  wires:
  Math Function1/1 -> Out2/1
  In1/1 -> Divide/1, Math Function/1
  Data Type Conversion/1 -> Out1/1
  1/1 -> Divide3/2
  Divide3/1 -> Divide2/2, Math Function1/2
  [ModeValue] -> Divide3/1
  In2/1 -> [ModeValue]
  Divide/1 -> Divide1/1
  [ModeValue] -> Divide/2
  [ModeValue] -> Math Function/2
  Sum1/1 -> Data Type Conversion/1
  Math Function/1 -> Math Function1/1, Divide2/1
  Divide1/1 -> Sum1/1
  7/1 -> Divide1/2
  Divide2/1 -> Sum1/2

== system ECO_TestLibs/LINASlave/Rx/Subsystem2/cntValue/ValueConvert2 ==
  In1 : Inport
  In2 : Inport  Port=2
  1 : Constant  Value=10  OutDataTypeStr=Inherit: Inherit via back propagation
  7 : Constant  Value=16  OutDataTypeStr=Inherit: Inherit via back propagation
  Data Type Conversion : DataTypeConversion
  Divide : Product  Inputs=*/
  Divide1 : Product  Inputs=**
  Divide2 : Product  Inputs=*/
  Divide3 : Product  Inputs=*/
  Math Function : Math  Operator=mod  SaturateOnIntegerOverflow=on
  Math Function1 : Math  Operator=mod  SaturateOnIntegerOverflow=on
  Sum1 : Sum  Inputs=|++
  Out1 : Outport
  Out2 : Outport  Port=2
  wires:
  Divide2/1 -> Sum1/2
  7/1 -> Divide1/2
  Divide1/1 -> Sum1/1
  Math Function/1 -> Divide2/1, Math Function1/1
  Sum1/1 -> Data Type Conversion/1
  [ModeValue] -> Math Function/2
  [ModeValue] -> Divide/2
  Divide/1 -> Divide1/1
  In2/1 -> [ModeValue]
  [ModeValue] -> Divide3/1
  Divide3/1 -> Math Function1/2, Divide2/2
  1/1 -> Divide3/2
  Data Type Conversion/1 -> Out1/1
  In1/1 -> Math Function/1, Divide/1
  Math Function1/1 -> Out2/1

== system ECO_TestLibs/LINASlave/Rx/Subsystem2/cntValue/ValueConvert3 ==
  In1 : Inport
  In2 : Inport  Port=2
  1 : Constant  Value=10  OutDataTypeStr=Inherit: Inherit via back propagation
  7 : Constant  Value=16  OutDataTypeStr=Inherit: Inherit via back propagation
  Data Type Conversion : DataTypeConversion
  Divide : Product  Inputs=*/
  Divide1 : Product  Inputs=**
  Divide2 : Product  Inputs=*/
  Divide3 : Product  Inputs=*/
  Math Function : Math  Operator=mod  SaturateOnIntegerOverflow=on
  Math Function1 : Math  Operator=mod  SaturateOnIntegerOverflow=on
  Sum1 : Sum  Inputs=|++
  Out1 : Outport
  Out2 : Outport  Port=2
  wires:
  Math Function1/1 -> Out2/1
  In1/1 -> Divide/1, Math Function/1
  Data Type Conversion/1 -> Out1/1
  1/1 -> Divide3/2
  Divide3/1 -> Divide2/2, Math Function1/2
  [ModeValue] -> Divide3/1
  In2/1 -> [ModeValue]
  Divide/1 -> Divide1/1
  [ModeValue] -> Divide/2
  [ModeValue] -> Math Function/2
  Sum1/1 -> Data Type Conversion/1
  Math Function/1 -> Math Function1/1, Divide2/1
  Divide1/1 -> Sum1/1
  7/1 -> Divide1/2
  Divide2/1 -> Sum1/2

== system ECO_TestLibs/LINASlave/Rx/Subsystem2/cntValue/ValueConvert4 ==
  In1 : Inport
  In2 : Inport  Port=2
  1 : Constant  Value=10  OutDataTypeStr=Inherit: Inherit via back propagation
  7 : Constant  Value=16  OutDataTypeStr=Inherit: Inherit via back propagation
  Data Type Conversion : DataTypeConversion
  Divide : Product  Inputs=*/
  Divide1 : Product  Inputs=**
  Divide2 : Product  Inputs=*/
  Divide3 : Product  Inputs=*/
  Math Function : Math  Operator=mod  SaturateOnIntegerOverflow=on
  Math Function1 : Math  Operator=mod  SaturateOnIntegerOverflow=on
  Sum1 : Sum  Inputs=|++
  Out1 : Outport
  Out2 : Outport  Port=2
  wires:
  Divide2/1 -> Sum1/2
  7/1 -> Divide1/2
  Divide1/1 -> Sum1/1
  Math Function/1 -> Divide2/1, Math Function1/1
  Sum1/1 -> Data Type Conversion/1
  [ModeValue] -> Math Function/2
  [ModeValue] -> Divide/2
  Divide/1 -> Divide1/1
  In2/1 -> [ModeValue]
  [ModeValue] -> Divide3/1
  Divide3/1 -> Math Function1/2, Divide2/2
  1/1 -> Divide3/2
  Data Type Conversion/1 -> Out1/1
  In1/1 -> Math Function/1, Divide/1
  Math Function1/1 -> Out2/1
